simulink model "nonlinear_controller"  (R2021a)
settings: Solver=FixedStepAuto  StartTime=0.0  StopTime=10.0  FixedStep=0.001  RelTol=1e-3
undefined symbols (not defined in the file): amplitude, offset, switch_degree
settings Model: OrderedModelArguments=off  Creator=chuanhui  LastModifiedBy=chuanhui

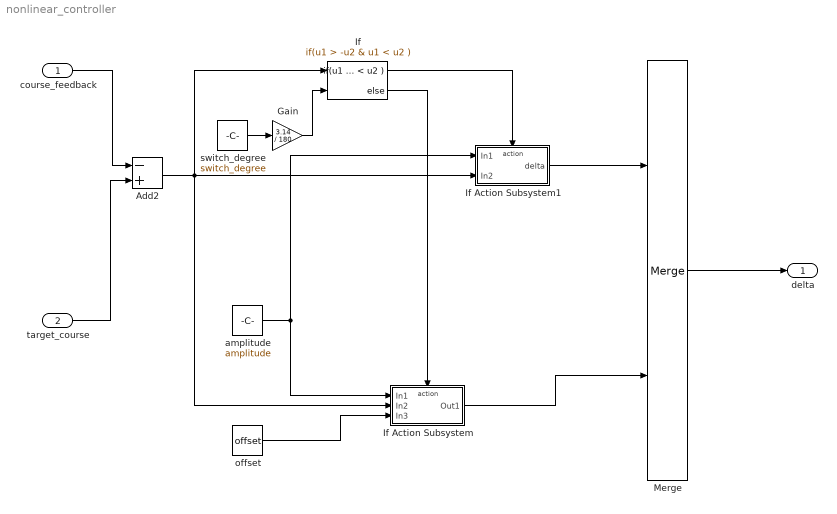
== system nonlinear_controller ==
  course_feedback : Inport
  target_course : Inport  Port=2
  Add2 : Sum  Inputs=-+
  Gain : Gain  Gain=3.14 / 180
  If : If  NumInputs=2  IfExpression=u1 > -u2 & u1 < u2
  If Action Subsystem : Subsystem  TreatAsAtomicUnit=on
  If Action Subsystem1 : Subsystem  TreatAsAtomicUnit=on
  Merge : Merge
  amplitude : Constant  Value=amplitude
  offset : Constant  Value=offset
  switch_degree : Constant  Value=switch_degree
  delta : Outport  Unit=rad/s  VectorParamsAs1DForOutWhenUnconnected=off
  wires:
  target_course/1 -> Add2/2
  course_feedback/1 -> Add2/1
  Add2/1 -> If Action Subsystem/2(In2), If Action Subsystem1/2(In2), If/1
  If/1 -> If Action Subsystem1/Action
  If/2 -> If Action Subsystem/Action
  amplitude/1 -> If Action Subsystem1/1(In1), If Action Subsystem/1(In1)
  offset/1 -> If Action Subsystem/3(In3)
  If Action Subsystem/1(Out1) -> Merge/2
  If Action Subsystem1/1(delta) -> Merge/1
  Merge/1 -> delta/1
  switch_degree/1 -> Gain/1
  Gain/1 -> If/2

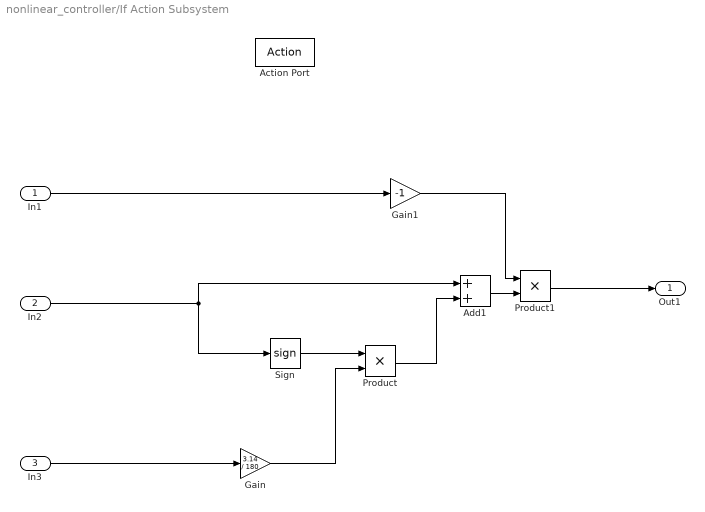
== system nonlinear_controller/If Action Subsystem ==
  In1 : Inport
  In2 : Inport  Port=2
  In3 : Inport  Port=3
  Action Port : ActionPort  ActionPortLabel=else
  Add1 : Sum
  Gain : Gain  Gain=3.14 / 180
  Gain1 : Gain  Gain=-1
  Product : Product
  Product1 : Product
  Sign : Signum
  Out1 : Outport
  wires:
  In2/1 -> Sign/1, Add1/1
  Add1/1 -> Product1/2
  Sign/1 -> Product/1
  In3/1 -> Gain/1
  Gain/1 -> Product/2
  Product/1 -> Add1/2
  Gain1/1 -> Product1/1
  In1/1 -> Gain1/1
  Product1/1 -> Out1/1

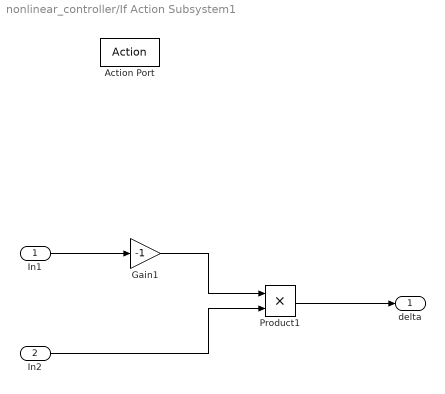
== system nonlinear_controller/If Action Subsystem1 ==
  In1 : Inport
  In2 : Inport  Port=2
  Action Port : ActionPort  ActionPortLabel=if(u1 > -u2 & u1 < u2 )
  Gain1 : Gain  Gain=-1
  Product1 : Product
  delta : Outport
  wires:
  Gain1/1 -> Product1/1
  In2/1 -> Product1/2
  Product1/1 -> delta/1
  In1/1 -> Gain1/1
